simulink model "BC_DC_MotorModel"  (R2022b)
settings: Solver=VariableStepAuto  StartTime=0.0  StopTime=10  RelTol=1e-3
undefined symbols (not defined in the file or in its folder): b, J, Ke, Kt, L, R
settings Model: Creator=altay  LastModifiedBy=aysen

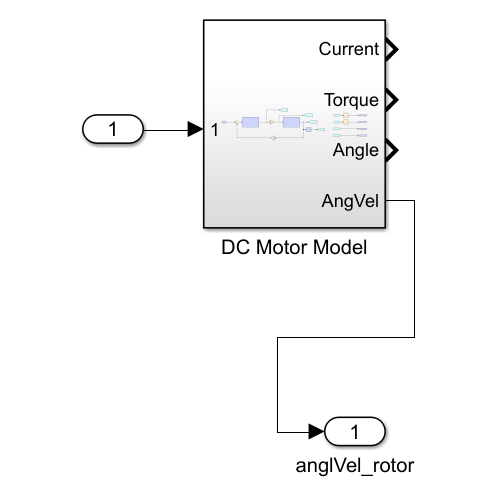
[thumbnail: Simulink's stored preview of the top-level diagram]
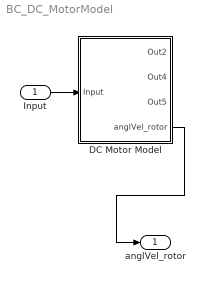
== system BC_DC_MotorModel ==
  Input : Inport
  DC Motor Model : Subsystem
  anglVel_rotor : Outport
  wires:
  DC Motor Model/4(anglVel_rotor) -> anglVel_rotor/1
  Input/1 -> DC Motor Model/1(Input)

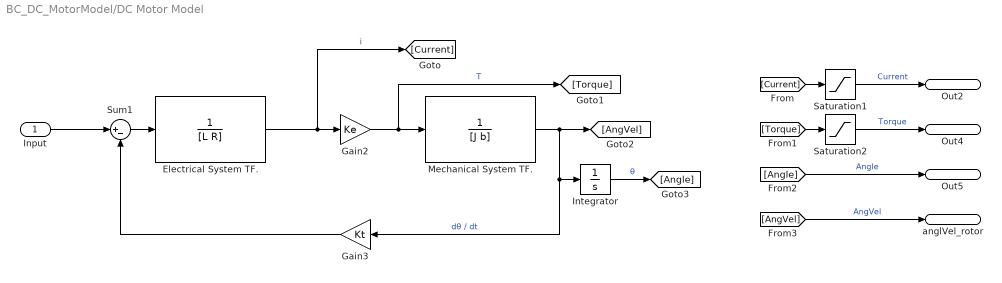
== system BC_DC_MotorModel/DC Motor Model ==
  Input : Inport
  Electrical System TF. : TransferFcn  Denominator=[L R]
  Gain2 : Gain  Gain=Ke
  Gain3 : Gain  Gain=Kt
  Integrator : Integrator
  Mechanical System TF. : TransferFcn  Denominator=[J b]
  Saturation1 : Saturate  UpperLimit=4.87  LowerLimit=-4.87
  Saturation2 : Saturate  UpperLimit=0.105  LowerLimit=-0.105
  Sum1 : Sum  Inputs=|+-
  Out2 : Outport
  Out4 : Outport  Port=2
  Out5 : Outport  Port=3
  anglVel_rotor : Outport  Port=4
  wires:
  Gain2/1 -> [Torque], Mechanical System TF./1  "T"
  Gain3/1 -> Sum1/2
  Electrical System TF./1 -> [Current], Gain2/1  "i"
  Sum1/1 -> Electrical System TF./1
  Input/1 -> Sum1/1
  Mechanical System TF./1 -> [AngVel], Integrator/1, Gain3/1  "dθ / dt"
  Integrator/1 -> [Angle]  "θ"
  Saturation1/1 -> Out2/1  "Current"
  [Current] -> Saturation1/1
  Saturation2/1 -> Out4/1  "Torque"
  [Torque] -> Saturation2/1
  [Angle] -> Out5/1  "Angle"
  [AngVel] -> anglVel_rotor/1  "AngVel"
